simulink library "Lib_Solve_Linearize_TMATS_org"  (Simulink 10.0)
settings: Solver=ode45  StartTime=0.0  StopTime=10.0  RelTol=1e-3  EnableMultiTasking=on
Description:
  | Thomas Modules
settings Model: Creator=jwchapm2  LastModifiedBy=bhisma

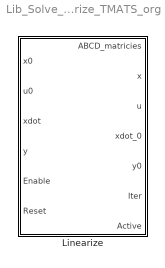
== system Lib_Solve_Linearize_TMATS_org ==
  Linearize : Subsystem  TreatAsAtomicUnit=on  mask(T-MATS: Linearize Library Block){N_XPer_M=[0.001 0.001], N_UPer_M=[0.001 0.001 0.001], N_Y_M=4}
      mask prompts: N_XPer_M "N_XPer_M - x Perturbation values (rxm)"; N_UPer_M "N_UPer_M - u Perturbation values (rxn)"; N_Y_M "N_Y_M - Number of expected y values (1x1)"
      mask help:
      | Determine State-space equation for a given system where:
      |
      | (xdot - xdot_0) = A*(x - x0) + B*(u - u0)
      | (y - y0) = C*(x - x0) + D*(u - u0)
      |
      | During operation each plant state (x) and input (u) will be set to an initial condition then perturbed separately. Perturbed inputs and system effects are compared against the baseline to determine the A,B,C, and D matricies. Perturbation sized are specified below. x0, u0, xdot_0, and y0 values are initial conditions. r is the number of perturbation per xdot or y.
      | Matrix sizes are specified as:
      | xdot and x : mx1
      | y : px1
      | u : nx1
      | A : mxm
      | B : mxn
      | C : pxm
      | D : pxn
      mask Help: web(which('Solver_TMATS_Linearize.html'),'-helpbrowser')

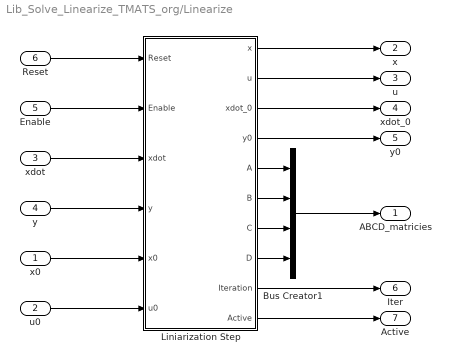
== system Lib_Solve_Linearize_TMATS_org/Linearize ==
  x0 : Inport
  u0 : Inport  Port=2
  xdot : Inport  Port=3
  y : Inport  Port=4
  Enable : Inport  Port=5
  Reset : Inport  Port=6
  Bus Creator1 : BusCreator  Inputs=4
  Liniarization Step : Subsystem  TreatAsAtomicUnit=on
  ABCD_matricies : Outport
  x : Outport  Port=2
  u : Outport  Port=3
  xdot_0 : Outport  Port=4
  y0 : Outport  Port=5
  Iter : Outport  Port=6
  Active : Outport  Port=7
  wires:
  Liniarization Step/4(y0) -> y0/1
  Liniarization Step/3(xdot_0) -> xdot_0/1
  Liniarization Step/10(Active) -> Active/1
  Liniarization Step/9(Iteration) -> Iter/1
  u0/1 -> Liniarization Step/6(u0)
  x0/1 -> Liniarization Step/5(x0)
  y/1 -> Liniarization Step/4(y)
  Liniarization Step/8(D) -> Bus Creator1/4
  Liniarization Step/7(C) -> Bus Creator1/3
  Liniarization Step/6(B) -> Bus Creator1/2
  Liniarization Step/5(A) -> Bus Creator1/1
  Liniarization Step/2("u ") -> u/1
  Liniarization Step/1(x) -> x/1
  Reset/1 -> Liniarization Step/1(Reset)
  Bus Creator1/1 -> ABCD_matricies/1
  xdot/1 -> Liniarization Step/3(xdot)
  Enable/1 -> Liniarization Step/2(Enable)

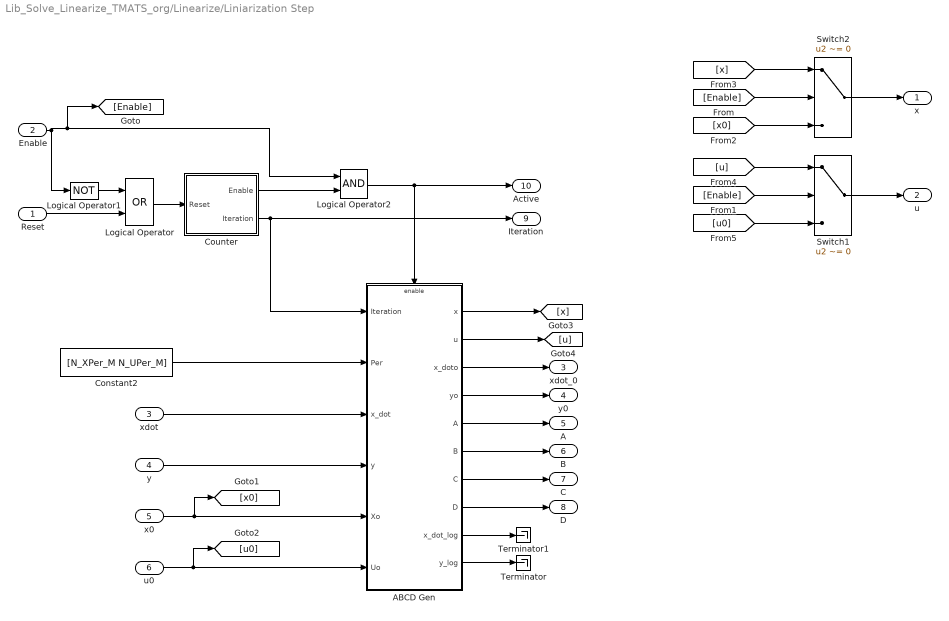
== system Lib_Solve_Linearize_TMATS_org/Linearize/Liniarization Step ==
  Reset : Inport
  Enable : Inport  Port=2
  xdot : Inport  Port=3
  y : Inport  Port=4
  x0 : Inport  Port=5
  u0 : Inport  Port=6
  ABCD Gen : Subsystem
  Constant2 : Constant  Value=[N_XPer_M N_UPer_M]
  Counter : Subsystem  mask{N_Ind_M=prod(size(N_XPer_M)) + prod(size(N_UPer_M))}
      mask prompts: N_Ind_M "number of independents, N_Ind_M"
  Logical Operator : Logic  Operator=OR  AllPortsSameDT=off  OutDataTypeStr=boolean
  Logical Operator1 : Logic  Operator=NOT  AllPortsSameDT=off  OutDataTypeStr=boolean
  Logical Operator2 : Logic  AllPortsSameDT=off  OutDataTypeStr=boolean
  Switch1 : Switch  Criteria=u2 ~= 0
  Switch2 : Switch  Criteria=u2 ~= 0
  Terminator : Terminator
  Terminator1 : Terminator
  x : Outport
  "u " : Outport  Port=2
  xdot_0 : Outport  Port=3
  y0 : Outport  Port=4
  A : Outport  Port=5
  B : Outport  Port=6
  C : Outport  Port=7
  D : Outport  Port=8
  Iteration : Outport  Port=9
  Active : Outport  Port=10
  wires:
  ABCD Gen/4(yo) -> y0/1
  ABCD Gen/3(x_doto) -> xdot_0/1
  ABCD Gen/6(B) -> B/1
  ABCD Gen/5(A) -> A/1
  ABCD Gen/2(u) -> [u]
  ABCD Gen/9(x_dot_log) -> Terminator1/1
  ABCD Gen/10(y_log) -> Terminator/1
  y/1 -> ABCD Gen/4(y)
  u0/1 -> [u0], ABCD Gen/6(Uo)
  xdot/1 -> ABCD Gen/3(x_dot)
  Constant2/1 -> ABCD Gen/2(Per)
  ABCD Gen/1(x) -> [x]
  Reset/1 -> Logical Operator/2
  Logical Operator2/1 -> ABCD Gen/Enable, Active/1
  x0/1 -> [x0], ABCD Gen/5(Xo)
  Counter/2(Iteration) -> Iteration/1, ABCD Gen/1(Iteration)
  ABCD Gen/8(D) -> D/1
  ABCD Gen/7(C) -> C/1
  Logical Operator/1 -> Counter/1(Reset)
  Logical Operator1/1 -> Logical Operator/1
  Counter/1(Enable) -> Logical Operator2/2
  Enable/1 -> [Enable], Logical Operator2/1, Logical Operator1/1
  [Enable] -> Switch2/2
  [Enable] -> Switch1/2
  Switch2/1 -> x/1
  Switch1/1 -> "u "/1
  [u] -> Switch1/1
  [u0] -> Switch1/3
  [x0] -> Switch2/3
  [x] -> Switch2/1

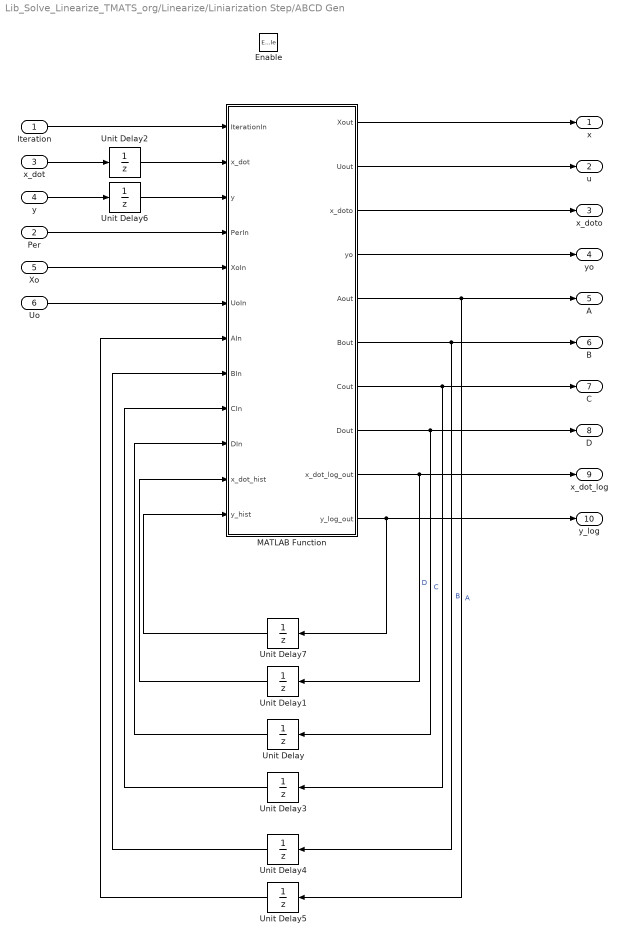
== system Lib_Solve_Linearize_TMATS_org/Linearize/Liniarization Step/ABCD Gen ==
  Iteration : Inport
  Per : Inport  Port=2
  x_dot : Inport  Port=3
  y : Inport  Port=4
  Xo : Inport  Port=5
  Uo : Inport  Port=6
  Enable : EnablePort
  MATLAB Function : MATLAB Function  TreatAsAtomicUnit=on
  Unit Delay : UnitDelay  InitialCondition=zeros(N_Y_M,size(N_UPer_M,2))  SampleTime=-1  HasFrameUpgradeWarning=on
  Unit Delay1 : UnitDelay  InitialCondition=zeros(size(N_XPer_M,2),prod(size(N_XPer_M))+prod(size(N_UPer_M))+1)  SampleTime=-1  HasFrameUpgradeWarning=on
  Unit Delay2 : UnitDelay  InitialCondition=zeros(size(N_XPer_M,2),1)  SampleTime=-1  HasFrameUpgradeWarning=on
  Unit Delay3 : UnitDelay  InitialCondition=zeros(N_Y_M,size(N_XPer_M,2))  SampleTime=-1  HasFrameUpgradeWarning=on
  Unit Delay4 : UnitDelay  InitialCondition=zeros(size(N_XPer_M,2),size(N_UPer_M,2))  SampleTime=-1  HasFrameUpgradeWarning=on
  Unit Delay5 : UnitDelay  InitialCondition=zeros(size(N_XPer_M,2),size(N_XPer_M,2))  SampleTime=-1  HasFrameUpgradeWarning=on
  Unit Delay6 : UnitDelay  InitialCondition=zeros(length(N_Y_M),1)  SampleTime=-1  HasFrameUpgradeWarning=on
  Unit Delay7 : UnitDelay  InitialCondition=zeros(N_Y_M,prod(size(N_XPer_M))+prod(size(N_UPer_M))+1)  SampleTime=-1  HasFrameUpgradeWarning=on
  x : Outport
  u : Outport  Port=2
  x_doto : Outport  Port=3
  yo : Outport  Port=4
  A : Outport  Port=5
  B : Outport  Port=6
  C : Outport  Port=7
  D : Outport  Port=8
  x_dot_log : Outport  Port=9
  y_log : Outport  Port=10
  wires:
  MATLAB Function/4(yo) -> yo/1
  MATLAB Function/3(x_doto) -> x_doto/1
  Unit Delay7/1 -> MATLAB Function/12(y_hist)
  y/1 -> Unit Delay6/1
  Unit Delay6/1 -> MATLAB Function/3(y)
  MATLAB Function/10(y_log_out) -> y_log/1, Unit Delay7/1
  MATLAB Function/2(Uout) -> u/1
  Uo/1 -> MATLAB Function/6(UoIn)
  Unit Delay5/1 -> MATLAB Function/7(AIn)
  Unit Delay4/1 -> MATLAB Function/8(BIn)
  Unit Delay3/1 -> MATLAB Function/9(CIn)
  Unit Delay/1 -> MATLAB Function/10(DIn)
  MATLAB Function/5(Aout) -> A/1, Unit Delay5/1  "A"
  MATLAB Function/6(Bout) -> Unit Delay4/1, B/1  "B"
  MATLAB Function/1(Xout) -> x/1
  Xo/1 -> MATLAB Function/5(XoIn)
  Per/1 -> MATLAB Function/4(PerIn)
  Iteration/1 -> MATLAB Function/1(IterationIn)
  MATLAB Function/7(Cout) -> C/1, Unit Delay3/1  "C"
  MATLAB Function/8(Dout) -> Unit Delay/1, D/1  "D"
  MATLAB Function/9(x_dot_log_out) -> Unit Delay1/1, x_dot_log/1
  Unit Delay1/1 -> MATLAB Function/11(x_dot_hist)
  x_dot/1 -> Unit Delay2/1
  Unit Delay2/1 -> MATLAB Function/2(x_dot)

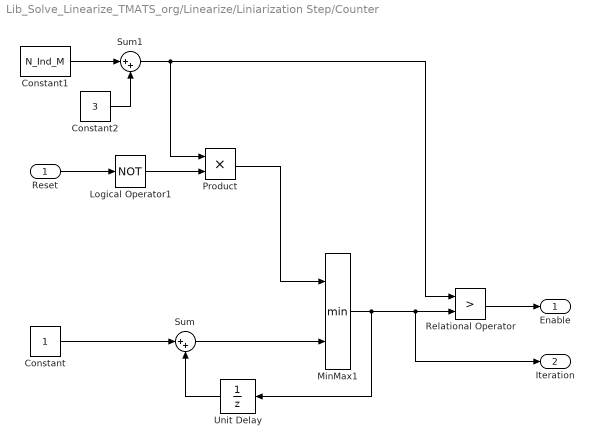
== system Lib_Solve_Linearize_TMATS_org/Linearize/Liniarization Step/Counter ==
  Reset : Inport
  Constant : Constant
  Constant1 : Constant  Value=N_Ind_M
  Constant2 : Constant  Value=3
  Logical Operator1 : Logic  Operator=NOT  AllPortsSameDT=off  OutDataTypeStr=boolean
  MinMax1 : MinMax  Inputs=2
  Product : Product  RndMeth=Zero
  Relational Operator : RelationalOperator  Operator=>  OutDataTypeStr=boolean  RndMeth=Nearest
  Sum : Sum  Inputs=|++
  Sum1 : Sum  Inputs=|++
  Unit Delay : UnitDelay  SampleTime=-1  HasFrameUpgradeWarning=on
  Enable : Outport
  Iteration : Outport  Port=2
  wires:
  Constant/1 -> Sum/1
  Product/1 -> MinMax1/1
  Sum/1 -> MinMax1/2
  Unit Delay/1 -> Sum/2
  MinMax1/1 -> Unit Delay/1, Iteration/1, Relational Operator/2
  Relational Operator/1 -> Enable/1
  Logical Operator1/1 -> Product/2
  Reset/1 -> Logical Operator1/1
  Sum1/1 -> Relational Operator/1, Product/1
  Constant2/1 -> Sum1/2
  Constant1/1 -> Sum1/1

== matlab function Linearize/Liniarization Step/ABCD Gen/MATLAB Function ==
  data: IterationIn input double; x_dot input double; y input double; PerIn input double; XoIn input double; UoIn input double; AIn input double; BIn input double; CIn input double; DIn input double; x_dot_hist input double; y_hist input double; Xout output double; Uout output double; x_doto output double; yo output double; Aout output double; Bout output double; Cout output double; Dout output double; x_dot_log_out output double; y_log_out output double
function [Xout, Uout,x_doto, yo, Aout, Bout, Cout, Dout, x_dot_log_out, y_log_out] = fcn(IterationIn, x_dot, y, PerIn, XoIn, UoIn, AIn, BIn, CIn, DIn, x_dot_hist, y_hist)
%Written by Jeffryes Chapman

% Set inital condiations
i = IterationIn;
Xout = XoIn;
Uout = UoIn;
XUmtrx = [Xout; Uout];
LenXU = length(XUmtrx);
LenX = length(Xout);
PerVec = reshape(PerIn.',1,[]);
LenPV = length(PerVec);
LenY = length(y);

%Check for matrix sizing
if length(x_dot) ~= LenX
    disp(' size of Xo does not match size of xdot');
end

% bring in ABCD matricies from memory
A = AIn;

% Inputing a 1 row matrix from simulink will be interpreted as a 1 col
% matrix in this matlab code. Flip matrixies if they meet the condition

if length(x_dot) == 1
    B = BIn';
    x_dot_log = x_dot_hist';
else
    B = BIn;
    x_dot_log = x_dot_hist;
end

if size(y_hist,2)==1
    C = CIn';
    D = DIn';
    y_log = y_hist';
else
    C = CIn;
    D = DIn;
    y_log = y_hist;
end

if size(PerIn,2)==1
    Per = PerIn';
else
    Per = PerIn;
end

% Begin taking data from f(x) at iteration a+1
a = 1;
% Begin determining ABCD Matricies at iteration b+1
b = a+1;

% Set Xout Output and Uout
if i > a && i <= LenPV + a
    % Determine XU value to be perturbed. May iterate through multiple
    % times if the Per matrix contains additional rows.
    current_XUnum = mod(i-a-1,LenXU)+1;
    % Perturb the X and U for determining output
    XUmtrx(current_XUnum) = XUmtrx(current_XUnum) + PerVec(i - a);
    % create output vectors
    Xout = XUmtrx(1:LenX);
    Uout = XUmtrx(LenX+1:LenXU);
end


% log x_dot and y values
if LenPV == 1
    if i == b;
        x_dot_log(1) = x_dot;
        y_log(1) = y;
    end
else
    if i > a && i<= LenPV + a+1;
        x_dot_log(:, i - a) = x_dot;
        y_log(:, i - a) = y;
    end
end

% Create ABCD matricies.
if i == LenPV + b
        % generate A&B matricies for all perturbation sets
        ABVec = (x_dot_log(:,2:end) - repmat(x_dot_log(:,1),1,LenPV))./repmat(PerVec,LenX,1);
        
        % Initialize sum matricies
        ABsum = zeros(LenX,LenXU);
        Nsum = zeros(LenX,LenXU);
        
        for set = 1: size(Per,1)
            % Determine current AB matrix to be analyzed
            AB_cur = ABVec(:, LenXU*(set-1)+1:LenXU*set);
            % Sum AB matrices for each set
            ABsum = ABsum + AB_cur(:,1:LenXU);
            % Sum number of acceptable values
            Nsum = Nsum + abs(sign(AB_cur(:,1:LenXU)));
        end
        
        % Average AB matricies for each perturbation set
        ABavg = ABsum./max(Nsum,1);
        
        % Separate A and B matricies
        A = ABavg(:,1:LenX);
        B = ABavg(:,LenX+1 :LenXU);
        
    % generate C&D matricies for each perturbation set
        CDVec = (y_log(:,2:end) - repmat(y_log(:,1),1,LenPV))./repmat(PerVec,LenY,1);
        

        % Initialize sum matricies
        CDsum = zeros(LenY,LenXU);
        NYsum = zeros(LenY,LenXU);
        
        for set = 1: size(Per,1)
            % Determine current CD matrix to be analyzed
            CD_cur = CDVec(:, LenXU*(set-1)+1:LenXU*set);
            % Sum CD matrices for each set
            CDsum = CDsum + CD_cur(:,1:LenXU);
            % Sum number of acceptable values
            NYsum = NYsum + abs(sign(CD_cur(:,1:LenXU)));
        end
        
        % Average CD matricies for each perturbation set
        CDavg = CDsum./max(NYsum,1);
        
        % Separate A and B matricies
        C = CDavg(:,1:LenX);
        D = CDavg(:,LenX+1 :LenXU);
end

x_doto = x_dot_log(:,1);
yo = y_log(:,1);

% Inputing a 1 row matrix from simulink will be interpreted as a 1 col
% matrix in this matlab code. Flip matrixies for output if they meet the condition.

Aout = A;
if length(x_dot) == 1
    Bout = B';
    x_dot_log_out = x_dot_log';
else
    Bout = B;
    x_dot_log_out = x_dot_log;
end

if size(y_hist,2)==1
    Cout = C';
    Dout = D';
    y_log_out = y_log';
else
    Cout = C;
    Dout = D;
    y_log_out = y_log;
end
